simulink model "auv_modell_camsim_controller"  (Simulink 7.0)
settings: Solver=ode45  StartTime=0.0  StopTime=1000  FixedStep=0.1  RelTol=1e-3
values from neighbouring files (symbols this model uses):
  eta0 = [-10 -5 6 0 0 0]'    [initauv.m]
undefined symbols (not defined in the file or in its folder): C_calc
libraries: marine_gnc x3, simulink_extras x3, simulink x1
settings Model: Creator=anderga  LastModifiedBy=anderga  BufferReuse=off
settings OptimizationCC: BlockReduction=off  InlineParams=on  BufferReuse=off

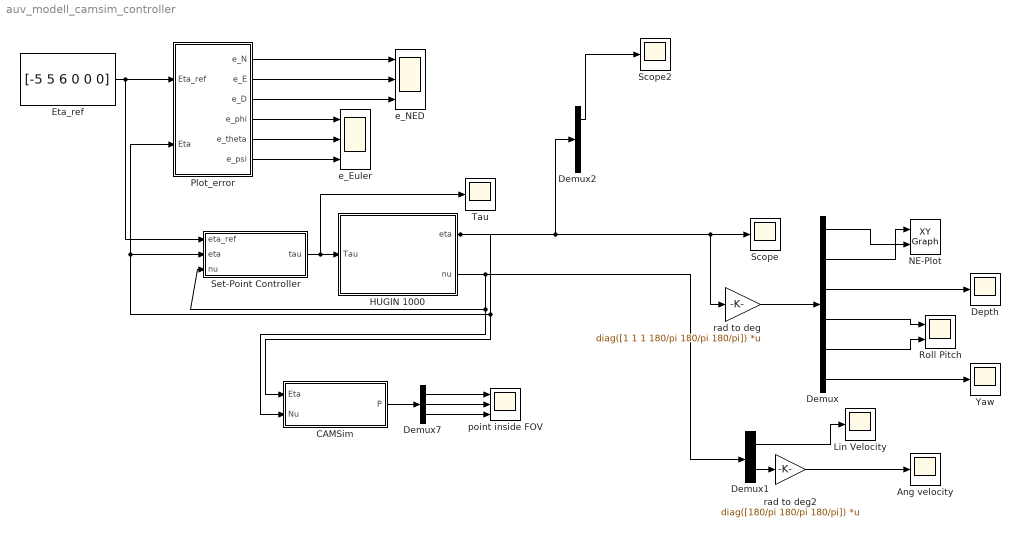
== system auv_modell_camsim_controller ==
  Ang velocity : Scope
      settings: YMin=-0.00015  YMax=0.00015  SaveName=ScopeData6
  CAMSim : Subsystem
  Demux : Demux  Outputs=6
  Demux1 : Demux  Outputs=2
  Demux2 : Demux  Outputs=3
  Demux7 : Demux  Outputs=3
  Depth : Scope
      settings: TimeRange=400  YMin=5  YMax=5.08  SaveName=ScopeData4
  Eta_ref : Constant  Value=[-5 5 6 0 0 0]  OutDataType=sfix(16)  OutScaling=2^0
  HUGIN 1000 : Subsystem  mask(HUGIN 1000 AUV){eta_0=eta0, nu_0=[0 0 0 0 0 0]}
      mask prompts: eta_0 "Initial Position [x y z phi theta psi]"; nu_0 "Initial speed [u v w p q r]"
      mask help:
      | The hydrodynamic model of Kongsberg Maritimes
      | AUV type HUGIN 1000.
      |
      | Implemented using
      |
      | eta_dot = J(eta)*nu
      | M*nu_dot + C(nu)*nu + D(nu)*nu + g(eta) = tau
      |
      | and the MMS toolbox from www.marinecybernetics.org
      mask init:
      | m = 1380;
      | xg = 0;
      | yg = 0;
      | zg = 0.0328;
      | Ix = 86.53;
      | Iy = 1247;
      | Iz = 1247;
      | 
      | Xu = -85.57;
      | Yv = -1092.9;
      | Yr = -84.1448;
      | Zw = -1092.9;
      | Zq = 84.1448;
      | Mq = -795.1686;
      | Nr = -795.1686;
      |     
      | M = [m-Xu   0       0       0       m*zg    -m*yg;
      |      0      m-Yv    0       -m*zg   0       m*xg-Yr;
      |      0      0       m-Zw    m*yg    -m*xg-Zq 0;
      |      0      -m*zg   m*yg    Ix      0        0;
      |      m*zg   0       -m*xg-Zq 0      Iy-Mq    0;
      |      -m*yg  m*xg-Yr 0       0       0       Iz-Nr];
  Lin Velocity : Scope
      settings: YMin=-1e-005  YMax=2.25e-005
  NE-Plot : simulink/Sinks/XY Graph  SystemSampleTime=-1  xmin=-100  xmax=220  ymin=-100  ymax=100  st=-1
  Plot_error : Subsystem
  Roll Pitch : Scope  NumInputPorts=2
      settings: TimeRange=400  YMin=-0.12~-0.01  YMax=0~0.05  SaveName=ScopeData3
  Scope : Scope
      settings: YMin=-12.5  YMax=7.5
  Scope2 : Scope
      settings: YMin=-10  YMax=10  SaveName=ScopeData10
  Set-Point Controller : Subsystem
  Tau : Scope
      settings: YMin=-100  YMax=100  SaveName=ScopeData11
  Yaw : Scope
      settings: TimeRange=100  YMin=45  YMax=45  SaveName=ScopeData2
  e_Euler : Scope  NumInputPorts=3
      settings: TimeRange=1000  YMin=-0.075~-0.5~-30  YMax=0.1~4~0  SaveName=ScopeData13
  e_NED : Scope  NumInputPorts=3
      settings: TimeRange=1000  YMin=-10~-5~5  YMax=-4~7.5~6.5  SaveName=ScopeData12
  point inside FOV : Scope  NumInputPorts=3
      settings: YMin=-9~-8~-8  YMax=4~6~6  SaveName=ScopeData9
  rad to deg : Gain  Gain=diag([1 1 1 180/pi 180/pi 180/pi])  Multiplication=Matrix(K*u)  ParameterDataType=sfix(16)  ParameterScaling=2^0  OutDataType=sfix(16)  OutScaling=2^0
  rad to deg2 : Gain  Gain=diag([180/pi 180/pi 180/pi])  Multiplication=Matrix(K*u)  ParameterDataType=sfix(16)  ParameterScaling=2^0  OutDataType=sfix(16)  OutScaling=2^0
  wires:
  HUGIN 1000/1(eta) -> rad to deg/1, Scope/1, Demux2/1, CAMSim/1(Eta), Set-Point Controller/2(eta), Plot_error/2(Eta)
  Demux/2 -> NE-Plot/1
  Demux/1 -> NE-Plot/2
  Demux/6 -> Yaw/1
  Demux/4 -> Roll Pitch/1
  Demux/5 -> Roll Pitch/2
  Demux/3 -> Depth/1
  Demux1/1 -> Lin Velocity/1
  Demux1/2 -> rad to deg2/1
  HUGIN 1000/2(nu) -> Demux1/1, CAMSim/2(Nu), Set-Point Controller/3(nu)
  rad to deg/1 -> Demux/1
  rad to deg2/1 -> Ang velocity/1
  Demux2/1 -> Scope2/1
  Set-Point Controller/1(tau) -> HUGIN 1000/1(Tau), Tau/1
  Eta_ref/1 -> Set-Point Controller/1(eta_ref), Plot_error/1(Eta_ref)
  CAMSim/1(P) -> Demux7/1
  Demux7/1 -> point inside FOV/1
  Demux7/2 -> point inside FOV/2
  Demux7/3 -> point inside FOV/3
  Plot_error/1(e_N) -> e_NED/1
  Plot_error/2(e_E) -> e_NED/2
  Plot_error/3(e_D) -> e_NED/3
  Plot_error/4(e_phi) -> e_Euler/1
  Plot_error/5(e_theta) -> e_Euler/2
  Plot_error/6(e_psi) -> e_Euler/3

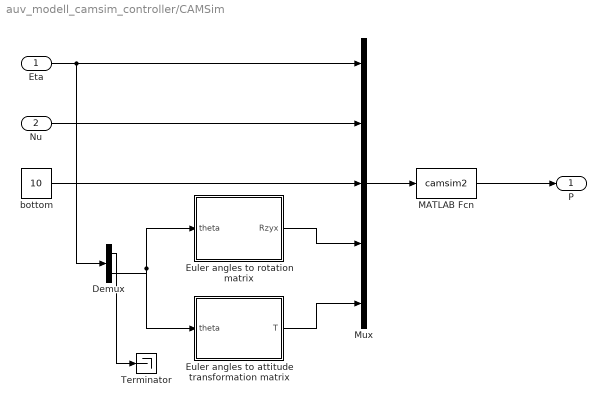
== system auv_modell_camsim_controller/CAMSim ==
  Eta : Inport  OutDataType=sfix(16)  OutScaling=2^0
  Nu : Inport  Port=2  OutDataType=sfix(16)  OutScaling=2^0
  Demux : Demux  Outputs=2
  Euler angles to rotation matrix : Subsystem  AncestorBlock=marine_gnc/Models/ Kinematics/Euler angles to rotation matrix
      mask Type: Euler2R
      mask Description:
      | Determine the 3-by-3 rotation matrix from the Euler angles (roll, pitch, yaw) using the zyx convention.
      | 
      | Output is a 9x1 vector
      mask Display:
      | port_label('input',1,'theta')
      | port_label('output',1,'R')
  Euler angles to attitude transformation matrix : Subsystem  AncestorBlock=marine_gnc/Models/ Kinematics/Euler angles to attitude transformation matrix
      mask Type: Euler2T
      mask Description: Determine the 3-by-3 attitude transformation matrix  from the Euler angles (roll, pitch, yaw).
      mask Display:
      | port_label('input',1,'theta')
      | port_label('output',1,'T')
  MATLAB Fcn : MATLABFcn  MATLABFcn=camsim2  OutputDimensions=6
  Mux : Mux  Inputs=5
  Terminator : Terminator
  bottom : Constant  Value=10  OutDataType=sfix(16)  OutScaling=2^0
  P : Outport  OutDataType=sfix(16)  OutScaling=2^0
  wires:
  Eta/1 -> Mux/1, Demux/1
  Nu/1 -> Mux/2
  bottom/1 -> Mux/3
  Mux/1 -> MATLAB Fcn/1
  MATLAB Fcn/1 -> P/1
  Demux/2 -> Euler angles to attitude transformation matrix/1(theta), Euler angles to rotation matrix/1(theta)
  Demux/1 -> Terminator/1
  Euler angles to rotation matrix/1(Rzyx) -> Mux/4
  Euler angles to attitude transformation matrix/1(T) -> Mux/5

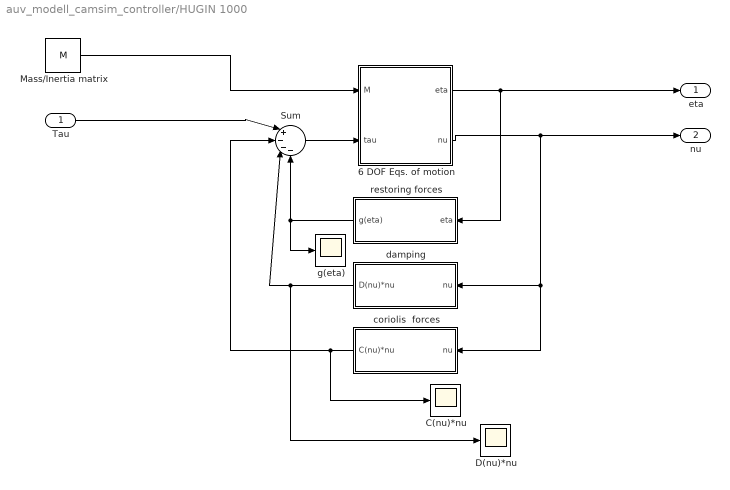
== system auv_modell_camsim_controller/HUGIN 1000 ==
  Tau : Inport  OutDataType=sfix(16)  OutScaling=2^0
  6 DOF Eqs. of motion : Subsystem  AncestorBlock=marine_gnc/Models/ Kinetics /6 DOF Eqs. of motion  mask(Equations of motion){nu0=nu_0, eta0=eta_0}
      mask prompts: nu0 "Initial velocities (u,v,w,p,q,r)"; eta0 "Initial position/attitude (x,y,z,phi,theta,psi)"
      mask help:
      | 6 DOF equations of motion (surge, sway, heave, roll, pitch and yaw)
      |
      |    eta_dot = J(eta)*nu
      |    (M_RB+M_A)*nu_dot  =  tau
      |
      | where nu = [u,v,w,p,q,r]'  and eta = [x,y,z,phi,theta,psi]'
      |
      | T. I. Fossen (2002). Marine Control Systems: Guidance, Navigation and Control of Ships, Rigs and Underwater Vehicles, Marine Cybernetics AS, ISBN 82-92356-00-2
      |
      | Modified by Anders Garmo (2008)
  C(nu)*nu : Scope
      settings: TimeRange=100  YMin=-0.1  YMax=1.2  SaveName=ScopeData5
  D(nu)*nu : Scope
      settings: TimeRange=100  YMin=-10  YMax=100  SaveName=ScopeData8
  Mass/Inertia matrix : Constant  Value=M  OutDataType=sfix(16)  OutScaling=2^0
  Sum : Sum  Inputs=|+---  OutDataType=sfix(16)  OutScaling=2^0
  coriolis  forces : Subsystem  Orientation=left
      mask init:
      | W = 1380*9.81;
      | 
      | zg = 0.0328;
  damping : Subsystem  Orientation=left
      mask init:
      | Xu = -19.1881;
      | Yv = -931.9715;
      | Yr = 1915.8;
      | Zw = -931.9715;
      | Zq = -1915.8;
      | Kp = -1000;
      | Mw = 1760.7;
      | Mq = -8386.3;
      | Nv = -1760.7;
      | Nr = -8386.3;
      | 
      | Xuu = -3.8938;
      | 
      | D = [Xu 0 0 0 0 0;
      |       0 Yv 0 0 0 Yr;
      |       0 0 Zw 0 Zq 0;
      |       0 0 0 Kp 0 0;
      |       0 0 Mw 0 Mq 0;
      |       0 Nv 0 0 0 Nr];
  g(eta) : Scope
      settings: TimeRange=100  YMin=0  YMax=100  SaveName=ScopeData7
  restoring forces : Subsystem  Orientation=left
      mask init:
      | W = 1380*9.81;
      | 
      | zg = 0.0328;
  eta : Outport  OutDataType=sfix(16)  OutScaling=2^0
  nu : Outport  Port=2  OutDataType=sfix(16)  OutScaling=2^0
  wires:
  Mass/Inertia matrix/1 -> 6 DOF Eqs. of motion/1(M)
  6 DOF Eqs. of motion/2(nu) -> nu/1, damping/1(nu), coriolis  forces/1(nu)
  6 DOF Eqs. of motion/1(eta) -> restoring forces/1(eta), eta/1
  Sum/1 -> 6 DOF Eqs. of motion/2(tau)
  Tau/1 -> Sum/1
  coriolis  forces/1(C(nu)*nu) -> C(nu)*nu/1, Sum/2
  restoring forces/1(g(eta)) -> Sum/4, g(eta)/1
  damping/1(D(nu)*nu) -> Sum/3, D(nu)*nu/1

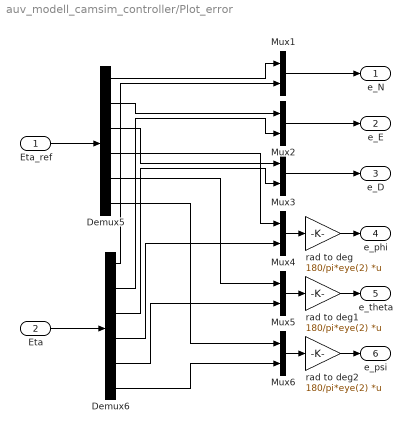
== system auv_modell_camsim_controller/Plot_error ==
  Eta_ref : Inport  OutDataType=sfix(16)  OutScaling=2^0
  Eta : Inport  Port=2  OutDataType=sfix(16)  OutScaling=2^0
  Demux5 : Demux  Outputs=6
  Demux6 : Demux  Outputs=6
  Mux{1..6} (6 alike) : Mux  Inputs=2
  rad to deg : Gain  Gain=180/pi*eye(2)  Multiplication=Matrix(K*u)  ParameterDataType=sfix(16)  ParameterScaling=2^0  OutDataType=sfix(16)  OutScaling=2^0
  rad to deg1 : Gain  Gain=180/pi*eye(2)  Multiplication=Matrix(K*u)  ParameterDataType=sfix(16)  ParameterScaling=2^0  OutDataType=sfix(16)  OutScaling=2^0
  rad to deg2 : Gain  Gain=180/pi*eye(2)  Multiplication=Matrix(K*u)  ParameterDataType=sfix(16)  ParameterScaling=2^0  OutDataType=sfix(16)  OutScaling=2^0
  e_N : Outport  OutDataType=sfix(16)  OutScaling=2^0
  e_E : Outport  Port=2  OutDataType=sfix(16)  OutScaling=2^0
  e_D : Outport  Port=3  OutDataType=sfix(16)  OutScaling=2^0
  e_phi : Outport  Port=4  OutDataType=sfix(16)  OutScaling=2^0
  e_theta : Outport  Port=5  OutDataType=sfix(16)  OutScaling=2^0
  e_psi : Outport  Port=6  OutDataType=sfix(16)  OutScaling=2^0
  wires:
  Demux5/1 -> Mux1/1
  Demux6/1 -> Mux1/2
  Demux5/2 -> Mux2/1
  Demux5/3 -> Mux3/1
  Demux6/2 -> Mux2/2
  Demux6/3 -> Mux3/2
  Eta/1 -> Demux6/1
  Mux1/1 -> e_N/1
  Mux2/1 -> e_E/1
  Mux3/1 -> e_D/1
  Mux4/1 -> rad to deg/1
  Mux5/1 -> rad to deg1/1
  Mux6/1 -> rad to deg2/1
  Demux5/4 -> Mux4/1
  Demux6/4 -> Mux4/2
  Demux5/5 -> Mux5/1
  Demux6/5 -> Mux5/2
  Demux6/6 -> Mux6/2
  Demux5/6 -> Mux6/1
  Eta_ref/1 -> Demux5/1
  rad to deg/1 -> e_phi/1
  rad to deg1/1 -> e_theta/1
  rad to deg2/1 -> e_psi/1

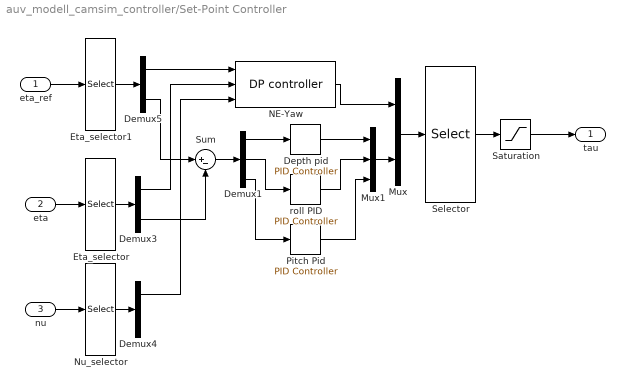
== system auv_modell_camsim_controller/Set-Point Controller ==
  eta_ref : Inport  OutDataType=sfix(16)  OutScaling=2^0
  eta : Inport  Port=2  OutDataType=sfix(16)  OutScaling=2^0
  nu : Inport  Port=3  OutDataType=sfix(16)  OutScaling=2^0
  Demux1 : Demux  Outputs=3
  Demux3 : Demux  Outputs=2
  Demux4 : Demux  Outputs=2
  Demux5 : Demux  Outputs=2
  Depth pid : simulink_extras/Additional Linear/PID Controller  SystemSampleTime=-1  P=50  I=1  D=0
  Eta_selector : Selector  InputPortWidth=6  IndexOptions=Index vector (dialog)  Indices=[1 2 6 3 4 5]  OutputSizes=1
  Eta_selector1 : Selector  InputPortWidth=6  IndexOptions=Index vector (dialog)  Indices=[1 2 6 3 4 5]  OutputSizes=1
  Mux : Mux  Inputs=2
  Mux1 : Mux  Inputs=3
  NE-Yaw : marine_gnc/Control/Dynamic  Positioning /DP controller  SystemSampleTime=-1  Kp=diag([230 300 1000])  Kd=diag([750 700 0])  Ki=diag([2 5 0])
  Nu_selector : Selector  InputPortWidth=6  IndexOptions=Index vector (dialog)  Indices=[1 2 6 3 4 5]  OutputSizes=1
  Pitch Pid : simulink_extras/Additional Linear/PID Controller  SystemSampleTime=-1  P=500  I=2  D=50
  Saturation : Saturate  UpperLimit=100  LowerLimit=-100  OutDataType=sfix(16)  OutScaling=2^0
  Selector : Selector  InputPortWidth=6  IndexOptions=Index vector (dialog)  Indices=[1 2 4 5 6 3]  OutputSizes=1
  Sum : Sum  Inputs=|+-  OutDataType=sfix(16)  OutScaling=2^0
  roll PID : simulink_extras/Additional Linear/PID Controller  SystemSampleTime=-1  P=0  I=0  D=0
  tau : Outport  OutDataType=sfix(16)  OutScaling=2^0
  wires:
  NE-Yaw/1 -> Mux/1
  Mux/1 -> Selector/1
  Mux1/1 -> Mux/2
  Eta_selector/1 -> Demux3/1
  Demux3/1 -> NE-Yaw/2
  Nu_selector/1 -> Demux4/1
  Demux4/1 -> NE-Yaw/3
  eta/1 -> Eta_selector/1
  nu/1 -> Nu_selector/1
  Selector/1 -> Saturation/1
  Saturation/1 -> tau/1
  eta_ref/1 -> Eta_selector1/1
  Demux5/2 -> Sum/1
  Demux5/1 -> NE-Yaw/1
  Eta_selector1/1 -> Demux5/1
  Demux3/2 -> Sum/2
  Sum/1 -> Demux1/1
  Demux1/1 -> Depth pid/1
  Depth pid/1 -> Mux1/1
  Demux1/2 -> roll PID/1
  roll PID/1 -> Mux1/2
  Demux1/3 -> Pitch Pid/1
  Pitch Pid/1 -> Mux1/3

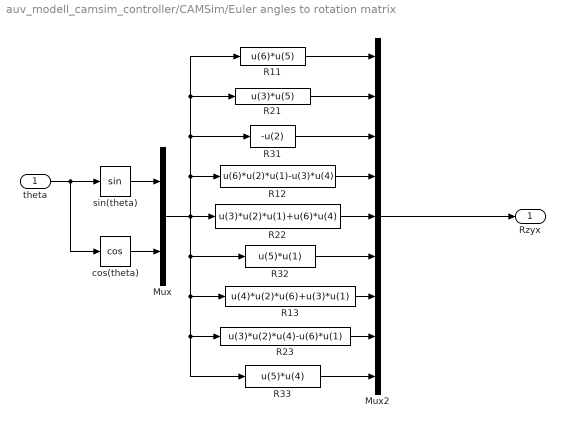
== system auv_modell_camsim_controller/CAMSim/Euler angles to rotation matrix ==
  theta : Inport  OutDataType=sfix(16)  OutScaling=2^0
  Mux : Mux  Inputs=2
  Mux2 : Mux  Inputs=9
  R11 : Fcn  Expr=u(6)*u(5)
  R12 : Fcn  Expr=u(6)*u(2)*u(1)-u(3)*u(4)
  R13 : Fcn  Expr=u(4)*u(2)*u(6)+u(3)*u(1)
  "R21 " : Fcn  Expr=u(3)*u(5)
  R22 : Fcn  Expr=u(3)*u(2)*u(1)+u(6)*u(4)
  R23 : Fcn  Expr=u(3)*u(2)*u(4)-u(6)*u(1)
  "R31 " : Fcn  Expr=-u(2)
  R32 : Fcn  Expr=u(5)*u(1)
  R33 : Fcn  Expr=u(5)*u(4)
  cos(theta) : Trigonometry  Operator=cos
  sin(theta) : Trigonometry
  Rzyx : Outport  OutDataType=sfix(16)  OutScaling=2^0  InitialOutput=0
  wires:
  R33/1 -> Mux2/9
  R32/1 -> Mux2/6
  "R21 "/1 -> Mux2/2
  "R31 "/1 -> Mux2/3
  R12/1 -> Mux2/4
  R22/1 -> Mux2/5
  R13/1 -> Mux2/7
  R23/1 -> Mux2/8
  Mux/1 -> R12/1, "R21 "/1, R11/1, "R31 "/1, R22/1, R23/1, R33/1, R13/1, R32/1
  theta/1 -> cos(theta)/1, sin(theta)/1
  cos(theta)/1 -> Mux/2
  sin(theta)/1 -> Mux/1
  Mux2/1 -> Rzyx/1
  R11/1 -> Mux2/1

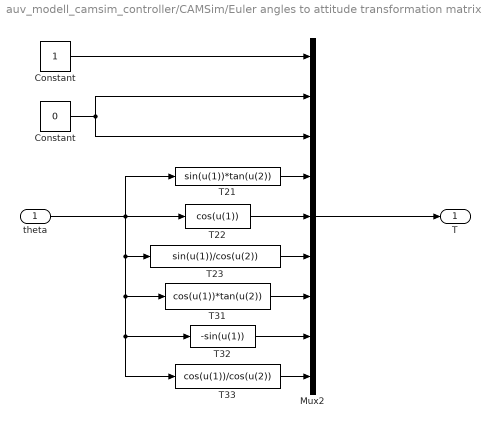
== system auv_modell_camsim_controller/CAMSim/Euler angles to attitude transformation matrix ==
  theta : Inport  OutDataType=sfix(16)  OutScaling=2^0
  Constant : Constant  OutDataType=sfix(16)  OutScaling=2^0
  "Constant " : Constant  Value=0  OutDataType=sfix(16)  OutScaling=2^0
  Mux2 : Mux  Inputs=9
  "T21 " : Fcn  Expr=sin(u(1))*tan(u(2))
  T22 : Fcn  Expr=cos(u(1))
  T23 : Fcn  Expr=sin(u(1))/cos(u(2))
  "T31 " : Fcn  Expr=cos(u(1))*tan(u(2))
  T32 : Fcn  Expr=-sin(u(1))
  T33 : Fcn  Expr=cos(u(1))/cos(u(2))
  T : Outport  OutDataType=sfix(16)  OutScaling=2^0  InitialOutput=0
  wires:
  T32/1 -> Mux2/8
  "T31 "/1 -> Mux2/7
  "T21 "/1 -> Mux2/4
  "Constant "/1 -> Mux2/3, Mux2/2
  T33/1 -> Mux2/9
  T22/1 -> Mux2/5
  T23/1 -> Mux2/6
  theta/1 -> "T21 "/1, T22/1, "T31 "/1, T32/1, T33/1, T23/1
  Mux2/1 -> T/1
  Constant/1 -> Mux2/1

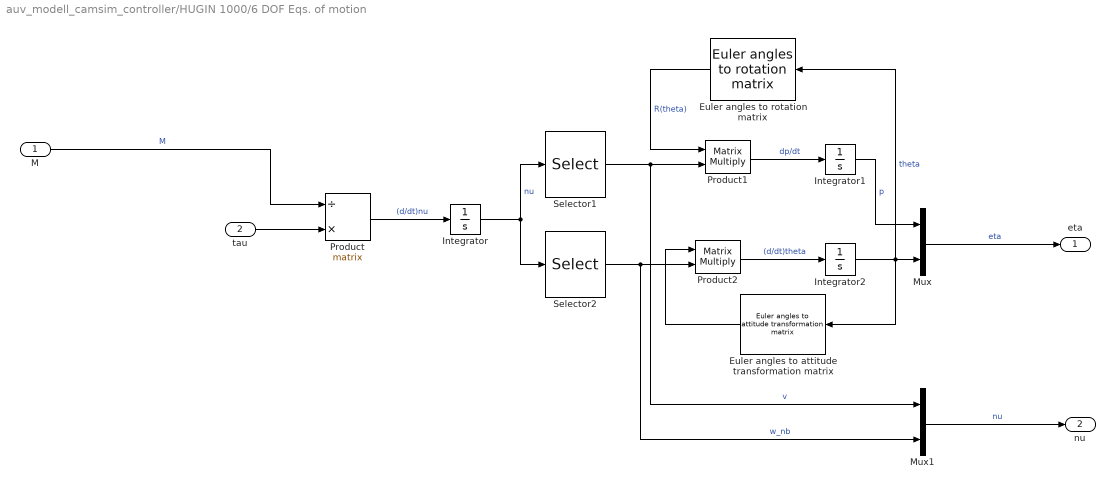
== system auv_modell_camsim_controller/HUGIN 1000/6 DOF Eqs. of motion ==
  M : Inport  OutDataType=sfix(16)  OutScaling=2^0
  tau : Inport  Port=2  OutDataType=sfix(16)  OutScaling=2^0
  Euler angles to rotation matrix : marine_gnc/Models/ Kinematics/Euler angles to rotation matrix  Orientation=left  SystemSampleTime=-1
  Euler angles to attitude transformation matrix : marine_gnc/Models/ Kinematics/Euler angles to attitude transformation matrix  Orientation=left  SystemSampleTime=-1
  Integrator : Integrator  InitialCondition=nu0
  Integrator1 : Integrator  InitialCondition=eta0(1:3)
  Integrator2 : Integrator  InitialCondition=eta0(4:6)
  Mux : Mux  Inputs=2
  Mux1 : Mux  Inputs=2
  Product : Product  Inputs=/*  Multiplication=Matrix(*)  OutDataType=sfix(16)  OutScaling=2^0  SaturateOnIntegerOverflow=on
  Product1 : Product  Inputs=**  Multiplication=Matrix(*)  OutDataType=sfix(16)  OutScaling=2^0  SaturateOnIntegerOverflow=on
  Product2 : Product  Inputs=**  Multiplication=Matrix(*)  OutDataType=sfix(16)  OutScaling=2^0  SaturateOnIntegerOverflow=on
  Selector1 : Selector  InputPortWidth=6  IndexOptions=Index vector (dialog)  Indices=[1 2 3]  OutputSizes=1
  Selector2 : Selector  InputPortWidth=6  IndexOptions=Index vector (dialog)  Indices=[4 5 6]  OutputSizes=1
  eta : Outport  OutDataType=sfix(16)  OutScaling=2^0
  nu : Outport  Port=2  OutDataType=sfix(16)  OutScaling=2^0
  wires:
  tau/1 -> Product/2
  Euler angles to attitude transformation matrix/1 -> Product2/1
  Mux1/1 -> nu/1  "nu"
  Mux/1 -> eta/1  "eta"
  Integrator1/1 -> Mux/1  "p"
  Integrator2/1 -> Euler angles to attitude transformation matrix/1, Euler angles to rotation matrix/1, Mux/2  "theta"
  Product2/1 -> Integrator2/1  "(d/dt)theta"
  Euler angles to rotation matrix/1 -> Product1/1  "R(theta)"
  Product1/1 -> Integrator1/1  "dp/dt"
  Selector2/1 -> Product2/2, Mux1/2  "w_nb"
  Selector1/1 -> Mux1/1, Product1/2  "v"
  Integrator/1 -> Selector2/1, Selector1/1  "nu"
  Product/1 -> Integrator/1  "(d/dt)nu"
  M/1 -> Product/1  "M"

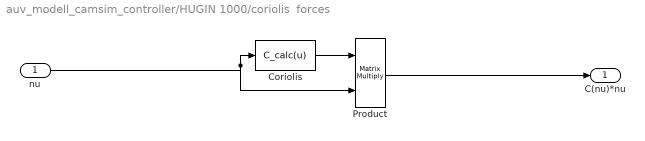
== system auv_modell_camsim_controller/HUGIN 1000/coriolis  forces ==
  nu : Inport  OutDataType=sfix(16)  OutScaling=2^0
  Coriolis : MATLABFcn  MATLABFcn=C_calc(u)  OutputDimensions=[6,6]  Output1D=off
  Product : Product  Multiplication=Matrix(*)  OutDataType=sfix(16)  OutScaling=2^0  RndMeth=Zero
  C(nu)*nu : Outport  OutDataType=sfix(16)  OutScaling=2^0
  wires:
  nu/1 -> Product/2, Coriolis/1
  Coriolis/1 -> Product/1
  Product/1 -> C(nu)*nu/1

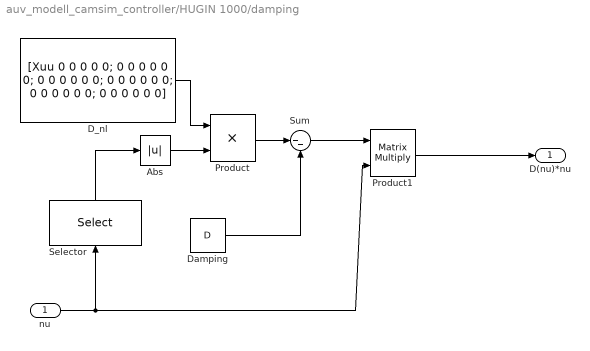
== system auv_modell_camsim_controller/HUGIN 1000/damping ==
  nu : Inport  OutDataType=sfix(16)  OutScaling=2^0
  Abs : Abs  OutDataType=sfix(16)  OutScaling=2^0
  D_nl : Constant  Value=[Xuu 0 0 0 0 0; 0 0 0 0 0 0; 0 0 0 0 0 0; 0 0 0 0 0 0; 0 0 0 0 0 0; 0 0 0 0 0 0]  OutDataType=sfix(16)  OutScaling=2^0
  Damping : Constant  Value=D  OutDataType=sfix(16)  OutScaling=2^0
  Product : Product  OutDataType=sfix(16)  OutScaling=2^0  RndMeth=Zero
  Product1 : Product  Multiplication=Matrix(*)  OutDataType=sfix(16)  OutScaling=2^0  RndMeth=Zero
  Selector : Selector  Orientation=up  InputPortWidth=6  IndexOptions=Index vector (dialog)  Indices=[1]  OutputSizes=1
  Sum : Sum  Inputs=|--  OutDataType=sfix(16)  OutScaling=2^0
  D(nu)*nu : Outport  OutDataType=sfix(16)  OutScaling=2^0
  wires:
  Damping/1 -> Sum/2
  Product/1 -> Sum/1
  nu/1 -> Product1/2, Selector/1
  D_nl/1 -> Product/1
  Abs/1 -> Product/2
  Sum/1 -> Product1/1
  Product1/1 -> D(nu)*nu/1
  Selector/1 -> Abs/1

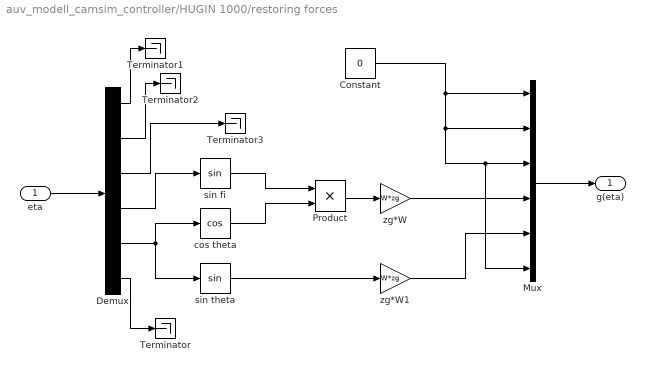
== system auv_modell_camsim_controller/HUGIN 1000/restoring forces ==
  eta : Inport  OutDataType=sfix(16)  OutScaling=2^0
  Constant : Constant  Value=0  OutDataType=sfix(16)  OutScaling=2^0
  Demux : Demux  Outputs=6
  Mux : Mux  Inputs=6
  Product : Product  OutDataType=sfix(16)  OutScaling=2^0  RndMeth=Zero
  Terminator{,1..3} (4 alike) : Terminator
  cos theta : Trigonometry  Operator=cos
  sin fi : Trigonometry
  sin theta : Trigonometry
  zg*W : Gain  Gain=W*zg  ParameterDataType=sfix(16)  ParameterScaling=2^0  OutDataType=sfix(16)  OutScaling=2^0
  zg*W1 : Gain  Gain=W*zg  ParameterDataType=sfix(16)  ParameterScaling=2^0  OutDataType=sfix(16)  OutScaling=2^0
  g(eta) : Outport  OutDataType=sfix(16)  OutScaling=2^0
  wires:
  eta/1 -> Demux/1
  Demux/4 -> sin fi/1
  Demux/5 -> cos theta/1, sin theta/1
  cos theta/1 -> Product/2
  sin fi/1 -> Product/1
  Product/1 -> zg*W/1
  sin theta/1 -> zg*W1/1
  Mux/1 -> g(eta)/1
  zg*W1/1 -> Mux/5
  zg*W/1 -> Mux/4
  Constant/1 -> Mux/1, Mux/2, Mux/3, Mux/6
  Demux/6 -> Terminator/1
  Demux/1 -> Terminator1/1
  Demux/2 -> Terminator2/1
  Demux/3 -> Terminator3/1
